simulink model "Tank_Backstepping_1_TIF"  (R2025b)
settings: Solver=ode45  StartTime=0.0  StopTime=250  RelTol=1e-3
model workspace (MAT data in the model file):
  Vp = Simulink.Parameter
  Vp.Complexity = 'real'
  Vp.Dimensions = [0 0]
  Vp.DataType = 'auto'
settings Model: Creator=juerg
settings DataIOCC: ReturnWorkspaceOutputs=off

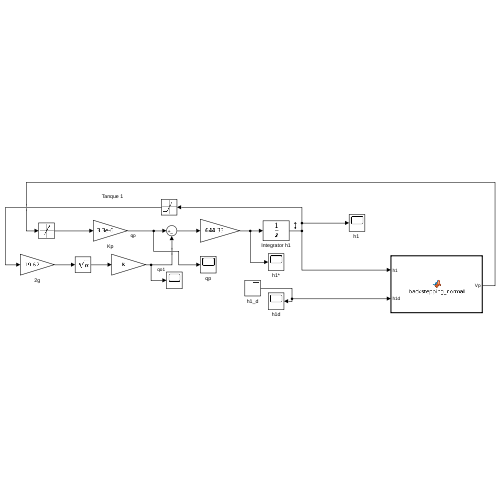
[thumbnail: Simulink's stored preview of the top-level diagram]
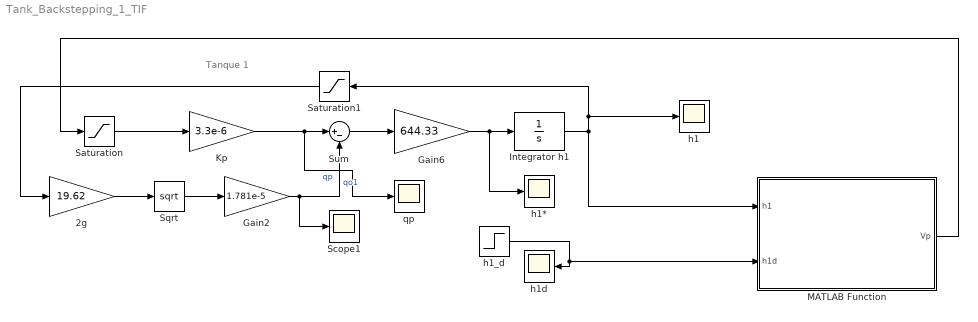
== system Tank_Backstepping_1_TIF ==
  note: Tanque 1
  2g : Gain  Gain=19.62
  Gain2 : Gain  Gain=1.781e-5
  Gain6 : Gain  Gain=644.33
  Integrator h1 : Integrator
  Kp : Gain  Gain=3.3e-6
  MATLAB Function : MATLAB Function  TreatAsAtomicUnit=on
  Saturation : Saturate  UpperLimit=10  LowerLimit=0
  Saturation1 : Saturate  UpperLimit=Inf  LowerLimit=0
  Scope1 : Scope
      settings: ActiveDisplayYMinimum=-8.5229773979433478E-6  ActiveDisplayYMaximum=7.6706796581490149E-5  DataLoggingVariableName=ScopeData5
  Sqrt : Sqrt
  Sum : Sum  Inputs=|+-
  "h1 " : Scope
      settings: ActiveDisplayYMinimum=-0.093378386042032  ActiveDisplayYMaximum=0.840405474378288
  h1* : Scope
      settings: ActiveDisplayYMinimum=-0.00549291325  ActiveDisplayYMaximum=0.04943621925000001  DataLoggingVariableName=ScopeData2
  h1_d : Step  Time=0.01  After=0.75  SampleTime=0
  h1d : Scope
      settings: ActiveDisplayYMinimum=-1  ActiveDisplayYMaximum=1  DataLoggingVariableName=ScopeData7
  qp : Scope
      settings: ActiveDisplayYMinimum=-8.5249999999999988E-6  ActiveDisplayYMaximum=7.6725000000000008E-5  DataLoggingVariableName=ScopeData4
  wires:
  2g/1 -> Sqrt/1
  Sqrt/1 -> Gain2/1
  Kp/1 -> qp/1, Sum/1  "qp"
  Gain2/1 -> Scope1/1, Sum/2  "qo1"
  Sum/1 -> Gain6/1
  Gain6/1 -> h1*/1, Integrator h1/1
  Saturation/1 -> Kp/1
  Saturation1/1 -> 2g/1
  MATLAB Function/1(Vp) -> Saturation/1
  Integrator h1/1 -> "h1 "/1, Saturation1/1, MATLAB Function/1(h1)
  h1_d/1 -> MATLAB Function/2(h1d), h1d/1

== matlab function Tank_Backstepping_1_TIF/MATLAB Function ==
  data: h1 input; Vp output; h1d input
function Vp = backstepping_normal(h1, h1d)
% --- Control Backstepping para UN solo tanque ---

% --- 1. Parámetros físicos del sistema ---
A1 = 1/644.33;        % Área del tanque 1 [m^2]
Cv1 = 1.781e-5;       % Coeficiente de descarga
c1 = 150;             % Ganancia del lazo interno

% Ganancia de la bomba (conocida)
Kp_conocido = 3.3e-6; 

% --- 2. Error de seguimiento ---
z1 = h1 - h1d;   % Error entre nivel actual y deseado

% --- 3. Ley de control Backstepping simplificada ---
% Dinámica del tanque: A1 * dh1/dt = Kp*Vp - Cv1*sqrt(h1)
% Control deseado: dh1/dt = -c1*z1
% Sustituyendo:
Vp = (A1 * (-c1 * z1) + Cv1 * sqrt(h1)) / Kp_conocido;

% --- 4. Saturación de la señal de control ---
Vp = min(max(Vp, 0.0), 10.0);

end
